simulink model "SMC"  (R2026a)
settings: Solver=VariableStepAuto
libraries: ros2lib x3
settings Model: Creator=hashaam1217  LastModifiedBy=hashaamzafar

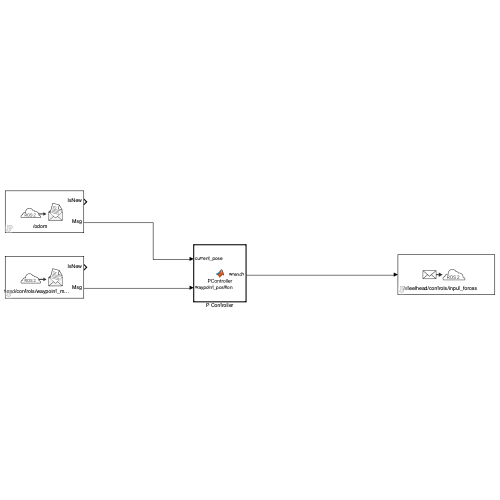
[thumbnail: Simulink's stored preview of the top-level diagram]
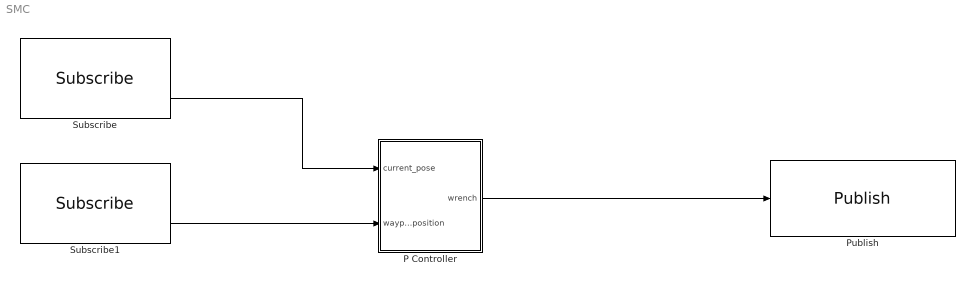
== system SMC ==
  P Controller : MATLAB Function  TreatAsAtomicUnit=on
  Publish : ros2lib/Publish  topicSource=Select from ROS network  topic=/steelhead/controls/input_forces  messageType=geometry_msgs/Wrench  QOSHistory=Keep last  QOSDepth=10  QOSReliability=Reliable  QOSDurability=Volatile  QOSDeadline=Inf  QOSLifespan=Inf  QOSLiveliness=Automatic  QOSLeaseDuration=Inf  QOSAvoidROSNamespaceConventions=off
  Subscribe : ros2lib/Subscribe  topicSource=Select from ROS network  topic=/odom  messageType=nav_msgs/Odometry  sampleTime=0.02  QOSHistory=Keep all  QOSDepth=10  QOSReliability=Reliable  QOSDurability=Volatile  QOSDeadline=Inf  QOSLifespan=Inf  QOSLiveliness=Automatic  QOSLeaseDuration=Inf  QOSAvoidROSNamespaceConventions=off
  Subscribe1 : ros2lib/Subscribe  topicSource=Select from ROS network  topic=/steelhead/controls/waypoint_marker/current_goal  messageType=geometry_msgs/Point  sampleTime=-1  QOSHistory=Keep last  QOSDepth=10  QOSReliability=Reliable  QOSDurability=Volatile  QOSDeadline=Inf  QOSLifespan=Inf  QOSLiveliness=Automatic  QOSLeaseDuration=Inf  QOSAvoidROSNamespaceConventions=off
  wires:
  Subscribe/2 -> P Controller/1(current_pose)
  P Controller/1(wrench) -> Publish/1
  Subscribe1/2 -> P Controller/2(waypoint_position)

== matlab function SMC/P Controller ==
  data: current_pose input; wrench output; waypoint_position input
function wrench = PController(current_pose, waypoint_position)
    % P Constants
    Kp_fx  = 100;
    Kp_fy  = 100;
    Kp_fz  = 100;
    Kp_yaw = 10;


    % Finding Error
    current_position = current_pose.position; 
    current_orientation = current_pose.orientation;
    vector_x = waypoint_position.x - current_position.x;
    vector_y = waypoint_position.y - current_position.y;
    vector_z = waypoint_position.z - current_position.z;

    error.yaw = atan2(vector_y, vector_x) - current_orientation;
    error.pose.yaw = mod(error.yaw + pi, 2*pi) - pi;
    error.pose.x   = vector_x;
    error.pose.y   = vector_y;
    error.pose.z   = vector_z;

    % In the format of geometry_msgs/Wrench.msg
    wrench = ros2('ros2msg', 'geometry_msgs/Wrench');

    % Applying P 
    wrench.force.x  = Kp_fx * error.pose.x;
    wrench.force.y  = Kp_fy * error.pose.y;
    wrench.force.z  = Kp_fz * error.pose.z;
    wrench.torque.x = 0;
    wrench.torque.y = 0;
    wrench.torque.z = Kp_yaw * error.pose.yaw;
end
